simulink model "modello_termico_a_blocchi"  (R2022b)
settings: Solver=VariableStepAuto  StartTime=0.0  StopTime=10000  RelTol=1e-3
values from neighbouring files (symbols this model uses):
  Cr = 0.1    [modello_termico.m]
  Cs = 100    [modello_termico.m]
  R1 = 1    [modello_termico.m]
  R2 = 10    [modello_termico.m]
settings Model: Creator=frvas  LastModifiedBy=frvas

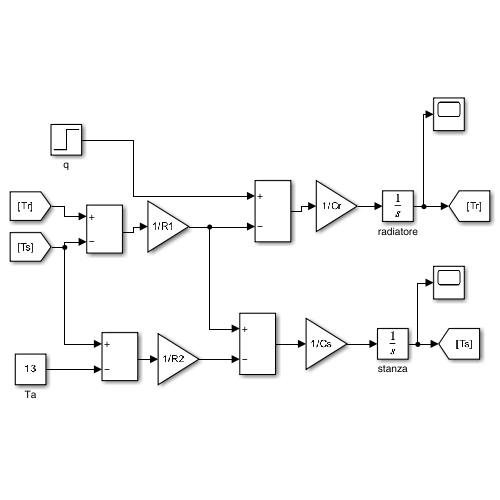
[thumbnail: Simulink's stored preview of the top-level diagram]
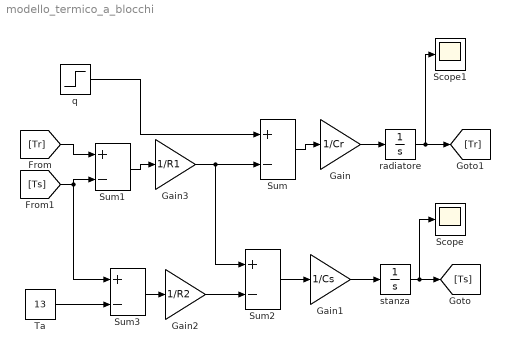
== system modello_termico_a_blocchi ==
  Gain : Gain  Gain=1/Cr
  Gain1 : Gain  Gain=1/Cs
  Gain2 : Gain  Gain=1/R2
  Gain3 : Gain  Gain=1/R1
  Scope : Scope
  Scope1 : Scope
  Sum{,1..3} (4 alike) : Sum  Inputs=+-
  Ta : Constant  Value=13
  q : Step  Time=250  SampleTime=0
  radiatore : Integrator  InitialCondition=20
  stanza : Integrator  InitialCondition=8
  wires:
  Gain/1 -> radiatore/1
  Gain1/1 -> stanza/1
  Sum/1 -> Gain/1
  stanza/1 -> Scope/1, [Ts]
  radiatore/1 -> Scope1/1, [Tr]
  Gain3/1 -> Sum2/1, Sum/2
  q/1 -> Sum/1
  [Tr] -> Sum1/1
  Sum1/1 -> Gain3/1
  [Ts] -> Sum3/1, Sum1/2
  Ta/1 -> Sum3/2
  Sum3/1 -> Gain2/1
  Gain2/1 -> Sum2/2
  Sum2/1 -> Gain1/1
